simulink model "FDIBenchMark_BLW_test_b_1025"  (Simulink 7.3)
settings: Solver=ode45  StartTime=0  StopTime=4400  FixedStep=Ts  RelTol=1e-12
InitFcn:
  | FDIBenchMarkData
  | initialization
values from neighbouring files (symbols this model uses):
  a = 2.2    [FDIBenchMarkData.m]
  Addt = [-(B_dt+B_r)/J_r B_dt/N_g/J_r -K_dt/J_r; eta_dt*B_dt/N_g/J_g -(eta_dt*B_dt/N_g^2+B_g)/J_g eta_dt*K_dt/N_g/J_g; 1 -1/N_g 0]    [FDIBenchMarkData.m]
  Addt2 = [-(B_dt+B_r)/J_r B_dt/N_g/J_r -K_dt/J_r; eta_dt2*B_dt/N_g/J_g -(eta_dt2*B_dt/N_g^2+B_g)/J_g eta_dt2*K_dt/N_g/J_g; 1 -1/N_g 0]    [FDIBenchMarkData.m]
  alpha = 0.1    [FDIBenchMarkData.m]
  alpha_gc = 1/20e-3    (= 50)    [FDIBenchMarkData.m]
  Apb_E = Apb+A_f    [initialization.m]
  Bddt = [1/J_r 0; 0 -1/J_g;0 0]    [FDIBenchMarkData.m]
  Bddt2 = [1/J_r 0; 0 -1/J_g;0 0]    [FDIBenchMarkData.m]
  Cddt = [1 0 0;0 1 0]    [FDIBenchMarkData.m]
  Constant_Beta_1_m1 = 5    [FDIBenchMarkData.m]
  Constant_Beta_3_m1 = 10    [FDIBenchMarkData.m]
  Constant_Omega_r_m1 = 1.4    [FDIBenchMarkData.m]
  Constant_tau_gc = 100    [FDIBenchMarkData.m]
  eta_gc = 0.98    [FDIBenchMarkData.m]
  Gain_Beta_2_m2 = 1.2    [FDIBenchMarkData.m]
  Gain_Omega_r_m2 = 1.1    [FDIBenchMarkData.m]
  H = 87    [FDIBenchMarkData.m]
  k = 4.7    [FDIBenchMarkData.m]
  K_i = 1    [FDIBenchMarkData.m]
  K_opt = .5* rho* pi*R^2*eta_dt*R^3*0.4554/(N_g*8)^3    (= 1.21708013189)    [FDIBenchMarkData.m]
  K_p = 4    [FDIBenchMarkData.m]
  L = Length_scale    (= 600)    [FDIBenchMarkData.m]
  Lpb = Lpb'    [initialization.m]
  Lpb_FD = Lpb_FD'    [initialization.m]
  m = 1+alpha*(alpha-1)*R^2/(8*H^2)    (= 0.995085835315)    [FDIBenchMarkData.m]
  m_vw = 1.5    [FDIBenchMarkData.m]
  Omega_delta = 15    [FDIBenchMarkData.m]
  omega_n = 11.11    [FDIBenchMarkData.m]
  Omega_nom = 162    [FDIBenchMarkData.m]
  P_r = 4.8e6    (= 4800000)    [FDIBenchMarkData.m]
  R = 57.5    [FDIBenchMarkData.m]
  r = D_rotor/2    (= 57.5)    [FDIBenchMarkData.m]
  r0 = 1.5    [FDIBenchMarkData.m]
  rho = 1.225    [FDIBenchMarkData.m]
  seed = ceil(seed)    [FDIBenchMarkData.m]
  T_sample = 0.05    [FDIBenchMarkData.m]
  Ts = 1/100    (= 0.01)    [FDIBenchMarkData.m]
  turb_int = Turbulence_intensity    (= 12)    [FDIBenchMarkData.m]
  turbulence_seeds = [seed1 seed2]    [FDIBenchMarkData.m]
  xi = 0.6    [FDIBenchMarkData.m]
undefined symbols (not defined in the file or in its folder): Apb, Apb1, Apb2, Bpb, Bpb1, Bpb2, Cpb, Cpb1, Cpb2, Cq, DiscIntNeverNeededParam, u0
libraries: simulink x30
(part 1 of 2)
settings Model: Creator=peodg  LastModifiedBy=WSUadm
settings SolverCC: MaxConsecutiveZCs=1e6
settings OptimizationCC: InitFltsAndDblsToZero=on

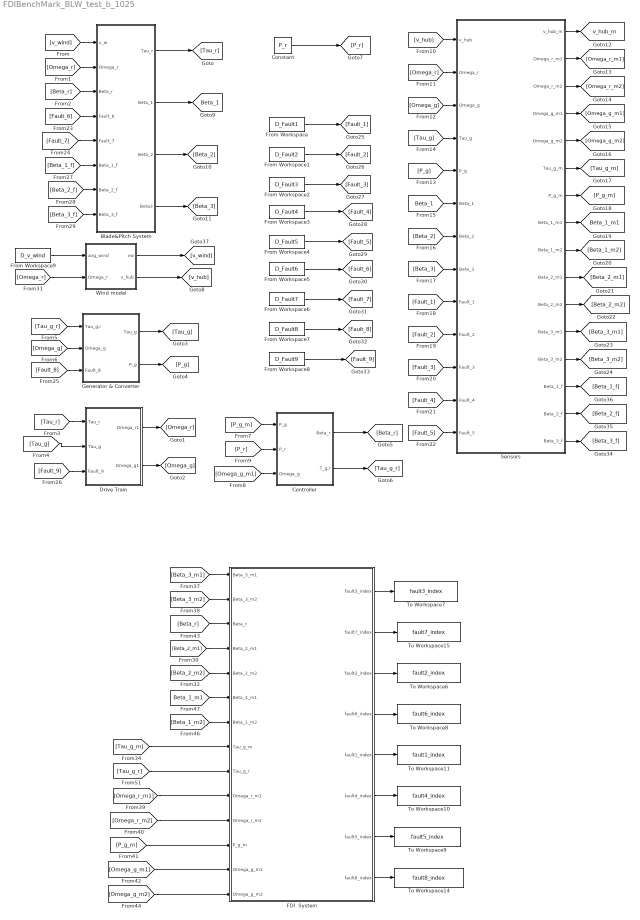
== system FDIBenchMark_BLW_test_b_1025 ==
  Blade&Pitch System : Subsystem
  Constant : Constant  Value=P_r  OutDataType=sfix(16)  OutScaling=2^0
  Controller : Subsystem
  Drive Train : Subsystem
  FDI  System : Subsystem
  From Workspace : FromWorkspace  VariableName=D_Fault1  SampleTime=Ts
  From Workspace1 : FromWorkspace  VariableName=D_Fault2  SampleTime=Ts
  From Workspace2 : FromWorkspace  VariableName=D_Fault3  SampleTime=Ts
  From Workspace3 : FromWorkspace  VariableName=D_Fault4  SampleTime=Ts
  From Workspace4 : FromWorkspace  VariableName=D_Fault5  SampleTime=Ts
  From Workspace5 : FromWorkspace  VariableName=D_Fault6  SampleTime=Ts
  From Workspace6 : FromWorkspace  VariableName=D_Fault7  SampleTime=Ts
  From Workspace7 : FromWorkspace  VariableName=D_Fault8  SampleTime=Ts
  From Workspace8 : FromWorkspace  VariableName=D_Fault9  SampleTime=Ts
  From Workspace9 : FromWorkspace  VariableName=D_v_wind
  Generator & Converter : Subsystem
  Sensors : Subsystem
  To Workspace10 : ToWorkspace  VariableName=fault4_index  SampleTime=-1  SaveFormat=Array
  To Workspace11 : ToWorkspace  VariableName=fault1_index  SampleTime=-1  SaveFormat=Array
  To Workspace14 : ToWorkspace  VariableName=fault8_index  SampleTime=-1  SaveFormat=Array
  To Workspace15 : ToWorkspace  VariableName=fault7_index  SampleTime=-1  SaveFormat=Array
  To Workspace6 : ToWorkspace  VariableName=fault2_index  SampleTime=-1  SaveFormat=Array
  To Workspace7 : ToWorkspace  VariableName=fault3_index  SampleTime=-1  SaveFormat=Array
  To Workspace8 : ToWorkspace  VariableName=fault6_index  SampleTime=-1  SaveFormat=Array
  To Workspace9 : ToWorkspace  VariableName=fault5_index  SampleTime=-1  SaveFormat=Array
  Wind model : Subsystem
  tag scope: Beta_1=global, Beta_1_m1=global, v_hub_m=global
  wires:
  [v_wind] -> Blade&Pitch System/1(v_w)
  [Omega_r] -> Blade&Pitch System/2(Omega_r)
  [Beta_r] -> Blade&Pitch System/3(Beta_r)
  [Tau_r] -> Drive Train/1(Tau_r)
  [Tau_g] -> Drive Train/2(Tau_g)
  Drive Train/1(Omega_r1) -> [Omega_r]
  [Tau_g_r] -> Generator & Converter/1(Tau_g,r)
  [Omega_g] -> Generator & Converter/2(Omega_g)
  Generator & Converter/1(Tau_g) -> [Tau_g]
  Generator & Converter/2(P_g) -> [P_g]
  [P_g_m] -> Controller/1(P_g)
  [Omega_g_m1] -> Controller/3(Omega_g)
  Controller/2(T_g,r) -> [Tau_g_r]
  [P_r] -> Controller/2(P_r)
  Constant/1 -> [P_r]
  Sensors/1(v_hub_m) -> [v_hub_m]
  Sensors/2(Omega_r_m1) -> [Omega_r_m1]
  Sensors/3(Omega_r_m2) -> [Omega_r_m2]
  Sensors/4(Omega_g_m1) -> [Omega_g_m1]
  Sensors/5(Omega_g_m2) -> [Omega_g_m2]
  Sensors/6(Tau_g_m) -> [Tau_g_m]
  Sensors/7(P_g_m) -> [P_g_m]
  Sensors/8(Beta_1_m1) -> [Beta_1_m1]
  Sensors/9(Beta_1_m2) -> [Beta_1_m2]
  Sensors/10(Beta_2_m1) -> [Beta_2_m1]
  Sensors/11(Beta_2_m2) -> [Beta_2_m2]
  Sensors/12(Beta_3_m1) -> [Beta_3_m1]
  Sensors/13(Beta_3_m2) -> [Beta_3_m2]
  [v_hub] -> Sensors/1(v_hub)
  [Omega_r] -> Sensors/2(Omega_r)
  [Omega_g] -> Sensors/3(Omega_g)
  [Tau_g] -> Sensors/4(Tau_g)
  [P_g] -> Sensors/5(P_g)
  [Beta_1] -> Sensors/6(Beta_1)
  [Beta_2] -> Sensors/7(Beta_2)
  [Beta_3] -> Sensors/8(Beta_3)
  [Fault_1] -> Sensors/9(Fault_1)
  [Fault_2] -> Sensors/10(Fault_2)
  [Fault_3] -> Sensors/11(Fault_3)
  [Fault_4] -> Sensors/12(Fault_4)
  [Fault_5] -> Sensors/13(Fault_5)
  [Fault_6] -> Blade&Pitch System/4(Fault_6)
  [Fault_7] -> Blade&Pitch System/5(Fault_7)
  [Fault_8] -> Generator & Converter/3(Fault_8)
  [Fault_9] -> Drive Train/3(Fault_9)
  From Workspace8/1 -> [Fault_9]
  From Workspace7/1 -> [Fault_8]
  From Workspace6/1 -> [Fault_7]
  From Workspace5/1 -> [Fault_6]
  From Workspace4/1 -> [Fault_5]
  From Workspace3/1 -> [Fault_4]
  From Workspace2/1 -> [Fault_3]
  From Workspace1/1 -> [Fault_2]
  From Workspace/1 -> [Fault_1]
  Drive Train/2(Omega_g1) -> [Omega_g]
  Sensors/16(Beta_3_f) -> [Beta_3_f]
  Sensors/15(Beta_2_f) -> [Beta_2_f]
  Sensors/14(Beta_1_f) -> [Beta_1_f]
  [Beta_1_f] -> Blade&Pitch System/6(Beta_1_f)
  [Beta_2_f] -> Blade&Pitch System/7(Beta_2_f)
  [Beta_3_f] -> Blade&Pitch System/8(Beta_3_f)
  Blade&Pitch System/4(Beta3) -> [Beta_3]
  Blade&Pitch System/3(Beta_2) -> [Beta_2]
  Blade&Pitch System/2(Beta_1) -> [Beta_1]
  Blade&Pitch System/1(Tau_r) -> [Tau_r]
  Wind model/1(vw) -> [v_wind]
  Wind model/2(v_hub) -> [v_hub]
  [Omega_r] -> Wind model/2(Omega_r)
  From Workspace9/1 -> Wind model/1(avg_wind)
  Controller/1(Beta_r) -> [Beta_r]
  FDI  System/1(fault3_index) -> To Workspace7/1
  FDI  System/2(fault7_index) -> To Workspace15/1
  [Beta_3_m1] -> FDI  System/1(Beta_3_m1)
  [Beta_3_m2] -> FDI  System/2(Beta_3_m2)
  FDI  System/3(fault2_index) -> To Workspace6/1
  FDI  System/4(fault6_index) -> To Workspace8/1
  [Beta_r] -> FDI  System/3(Beta_r)
  [Beta_2_m1] -> FDI  System/4(Beta_2_m1)
  [Beta_2_m2] -> FDI  System/5(Beta_2_m2)
  FDI  System/5(fault1_index) -> To Workspace11/1
  [Beta_1_m2] -> FDI  System/7(Beta_1_m2)
  [Beta_1_m1] -> FDI  System/6(Beta_1_m1)
  FDI  System/6(fault4_index) -> To Workspace10/1
  FDI  System/7(fault5_index) -> To Workspace9/1
  FDI  System/8(fault8_index) -> To Workspace14/1
  [Omega_g_m1] -> FDI  System/13(Omega_g_m1)
  [Omega_r_m1] -> FDI  System/10(Omega_r_m1)
  [Tau_g_m] -> FDI  System/8(Tau_g_m)
  [Omega_r_m2] -> FDI  System/11(Omega_r_m2)
  [Tau_g_r] -> FDI  System/9(Tau_g_r)
  [P_g_m] -> FDI  System/12(P_g_m)
  [Omega_g_m2] -> FDI  System/14(Omega_g_m2)

== system FDIBenchMark_BLW_test_b_1025/Blade&Pitch System ==
  v_w : Inport  OutDataType=sfix(16)  OutScaling=2^0
  Omega_r : Inport  Port=2  OutDataType=sfix(16)  OutScaling=2^0
  Beta_r : Inport  Port=3  OutDataType=sfix(16)  OutScaling=2^0
  Fault_6 : Inport  Port=4  OutDataType=sfix(16)  OutScaling=2^0
  Fault_7 : Inport  Port=5  OutDataType=sfix(16)  OutScaling=2^0
  Beta_1_f : Inport  Port=6  OutDataType=sfix(16)  OutScaling=2^0
  Beta_2_f : Inport  Port=7  OutDataType=sfix(16)  OutScaling=2^0
  Beta_3_f : Inport  Port=8  OutDataType=sfix(16)  OutScaling=2^0
  Add : Sum  OutDataType=sfix(16)  OutScaling=2^-10
  Add1 : Sum  OutDataType=sfix(16)  OutScaling=2^-10
  Add2 : Sum  OutDataType=sfix(16)  OutScaling=2^-10
  Pitch Systems : Subsystem
  Subsystem : Subsystem
  To Workspace6 : ToWorkspace  VariableName=Tau_r  SampleTime=-1  SaveFormat=Array
  Tau_r : Outport  OutDataType=sfix(16)  OutScaling=2^0
  Beta_1 : Outport  Port=2  OutDataType=sfix(16)  OutScaling=2^0
  Beta_2 : Outport  Port=3  OutDataType=sfix(16)  OutScaling=2^0
  Beta3 : Outport  Port=4  OutDataType=sfix(16)  OutScaling=2^0
  wires:
  Pitch Systems/1(Beta_1) -> Subsystem/3(Beta_1), Beta_1/1
  Pitch Systems/2(Beta_2) -> Subsystem/4(Beta_2), Beta_2/1
  Pitch Systems/3(Beta_3) -> Subsystem/5(Beta_3), Beta3/1
  Subsystem/1(Tau_r) -> Tau_r/1, To Workspace6/1
  v_w/1 -> Subsystem/1(v_w)
  Omega_r/1 -> Subsystem/2(Omega_r)
  Fault_6/1 -> Pitch Systems/4(Fault_6)
  Fault_7/1 -> Pitch Systems/5(Fault_7)
  Add/1 -> Pitch Systems/3(Beta_r3)
  Add1/1 -> Pitch Systems/1(Beta_r1)
  Add2/1 -> Pitch Systems/2(Beta_r2)
  Beta_3_f/1 -> Add/2
  Beta_2_f/1 -> Add2/2
  Beta_1_f/1 -> Add1/2
  Beta_r/1 -> Add1/1, Add2/1, Add/1

== system FDIBenchMark_BLW_test_b_1025/Controller ==
  P_g : Inport  OutDataType=sfix(16)  OutScaling=2^0
  P_r : Inport  Port=2  OutDataType=sfix(16)  OutScaling=2^0
  Omega_g : Inport  Port=3  OutDataType=sfix(16)  OutScaling=2^0
  Constant : Constant  Value=Omega_nom  OutDataType=sfix(16)  OutScaling=2^0
  Constant1 : Constant  Value=Omega_delta  OutDataType=sfix(16)  OutScaling=2^0
  Embedded MATLAB Function : Stateflow chart
  Subsystem : Subsystem
  Subsystem1 : Subsystem
  Switch : Switch  Threshold=.5  OutDataType=sfix(16)  OutScaling=2^0
  Switch1 : Switch  Threshold=.5  OutDataType=sfix(16)  OutScaling=2^0
  Unit Delay : UnitDelay  SampleTime=Ts
  Zero-Order Hold : ZeroOrderHold  SampleTime=Ts
  Zero-Order Hold1 : ZeroOrderHold  SampleTime=Ts
  Zero-Order Hold2 : ZeroOrderHold  SampleTime=Ts
  Beta_r : Outport  OutDataType=sfix(16)  OutScaling=2^0
  T_g,r : Outport  Port=2  OutDataType=sfix(16)  OutScaling=2^0
  wires:
  Embedded MATLAB Function/1(ControlZone) -> Unit Delay/1, Switch/2, Switch1/2
  Unit Delay/1 -> Embedded MATLAB Function/4(LastControlZone)
  P_g/1 -> Zero-Order Hold/1
  P_r/1 -> Zero-Order Hold1/1
  Omega_g/1 -> Zero-Order Hold2/1
  Switch/1 -> Beta_r/1
  Switch1/1 -> T_g,r/1
  Subsystem1/1(Beta_r) -> Switch/1
  Subsystem/1(Beta_r) -> Switch/3
  Subsystem1/2(Tau_g,r) -> Switch1/1
  Subsystem/2(T_g,r) -> Switch1/3
  Constant/1 -> Embedded MATLAB Function/5(Omega_nom)
  Constant1/1 -> Embedded MATLAB Function/6(Omega_delta)
  Zero-Order Hold/1 -> Embedded MATLAB Function/1(P_g)
  Zero-Order Hold1/1 -> Embedded MATLAB Function/2(P_r), Subsystem1/1(P_r)
  Zero-Order Hold2/1 -> Embedded MATLAB Function/3(Omega_g), Subsystem1/2(Omega_g), Subsystem/1(Omega_g)

== system FDIBenchMark_BLW_test_b_1025/Drive Train ==
  Tau_r : Inport  OutDataType=sfix(16)  OutScaling=2^0
  Tau_g : Inport  Port=2  OutDataType=sfix(16)  OutScaling=2^0
  Fault_9 : Inport  Port=3  OutDataType=sfix(16)  OutScaling=2^0
  Add : Sum  OutDataType=sfix(16)  OutScaling=2^-10
  Demux1 : Demux  Outputs=2
  Gain : Gain  Gain=Addt  Multiplication=Matrix(K*u)  ParameterDataType=sfix(16)  ParameterScaling=2^0  OutDataType=sfix(16)  OutScaling=2^0
  Gain1 : Gain  Gain=Bddt  Multiplication=Matrix(K*u)  ParameterDataType=sfix(16)  ParameterScaling=2^0  OutDataType=sfix(16)  OutScaling=2^0
  Gain2 : Gain  Gain=Cddt  Multiplication=Matrix(K*u)  ParameterDataType=sfix(16)  ParameterScaling=2^0  OutDataType=sfix(16)  OutScaling=2^0
  Gain3 : Gain  Gain=Addt2  Multiplication=Matrix(K*u)  ParameterDataType=sfix(16)  ParameterScaling=2^0  OutDataType=sfix(16)  OutScaling=2^0
  Gain4 : Gain  Gain=Bddt2  Multiplication=Matrix(K*u)  ParameterDataType=sfix(16)  ParameterScaling=2^0  OutDataType=sfix(16)  OutScaling=2^0
  Integrator : Integrator  InitialCondition=[1 100 0]
  Mux : Mux  Inputs=2
  Switch1 : Switch  Threshold=0.5  OutDataType=sfix(16)  OutScaling=2^0
  Switch2 : Switch  Threshold=0.5  OutDataType=sfix(16)  OutScaling=2^0
  Omega_r1 : Outport  OutDataType=sfix(16)  OutScaling=2^0
  Omega_g1 : Outport  Port=2  OutDataType=sfix(16)  OutScaling=2^0
  wires:
  Tau_r/1 -> Mux/1
  Tau_g/1 -> Mux/2
  Integrator/1 -> Gain/1, Gain3/1, Gain2/1
  Add/1 -> Integrator/1
  Switch1/1 -> Add/1
  Gain1/1 -> Switch1/1
  Gain4/1 -> Switch1/3
  Gain/1 -> Switch2/1
  Gain3/1 -> Switch2/3
  Switch2/1 -> Add/2
  Demux1/1 -> Omega_r1/1
  Demux1/2 -> Omega_g1/1
  Gain2/1 -> Demux1/1
  Fault_9/1 -> Switch1/2, Switch2/2
  Mux/1 -> Gain1/1, Gain4/1

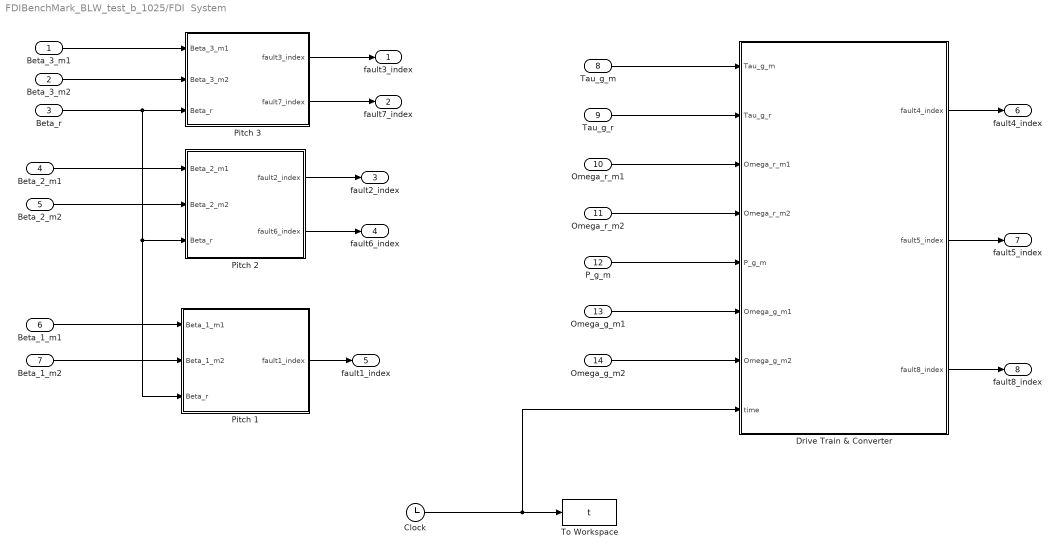
== system FDIBenchMark_BLW_test_b_1025/FDI  System ==
  Beta_3_m1 : Inport  OutDataType=fixdt(1, 16)  OutScaling=2^0
  Beta_3_m2 : Inport  Port=2  OutDataType=fixdt(1, 16)  OutScaling=2^0
  Beta_r : Inport  Port=3  OutDataType=fixdt(1, 16)  OutScaling=2^0
  Beta_2_m1 : Inport  Port=4  OutDataType=fixdt(1, 16)  OutScaling=2^0
  Beta_2_m2 : Inport  Port=5  OutDataType=fixdt(1, 16)  OutScaling=2^0
  Beta_1_m1 : Inport  Port=6  OutDataType=fixdt(1, 16)  OutScaling=2^0
  Beta_1_m2 : Inport  Port=7  OutDataType=fixdt(1, 16)  OutScaling=2^0
  Tau_g_m : Inport  Port=8  OutDataType=fixdt(1, 16)  OutScaling=2^0
  Tau_g_r : Inport  Port=9  OutDataType=fixdt(1, 16)  OutScaling=2^0
  Omega_r_m1 : Inport  Port=10  OutDataType=fixdt(1, 16)  OutScaling=2^0
  Omega_r_m2 : Inport  Port=11  OutDataType=fixdt(1, 16)  OutScaling=2^0
  P_g_m : Inport  Port=12  OutDataType=fixdt(1, 16)  OutScaling=2^0
  Omega_g_m1 : Inport  Port=13  OutDataType=fixdt(1, 16)  OutScaling=2^0
  Omega_g_m2 : Inport  Port=14  OutDataType=fixdt(1, 16)  OutScaling=2^0
  Clock : Clock
      settings: Decimation=10
  Drive Train & Converter : Subsystem
  Pitch 1 : Subsystem
  Pitch 2 : Subsystem
  Pitch 3 : Subsystem
  To Workspace : ToWorkspace  VariableName=t  SampleTime=-1  SaveFormat=Array
  fault3_index : Outport  OutDataType=fixdt(1, 16)  OutScaling=2^0
  fault7_index : Outport  Port=2  OutDataType=fixdt(1, 16)  OutScaling=2^0
  fault2_index : Outport  Port=3  OutDataType=fixdt(1, 16)  OutScaling=2^0
  fault6_index : Outport  Port=4  OutDataType=fixdt(1, 16)  OutScaling=2^0
  fault1_index : Outport  Port=5  OutDataType=fixdt(1, 16)  OutScaling=2^0
  fault4_index : Outport  Port=6  OutDataType=fixdt(1, 16)  OutScaling=2^0
  fault5_index : Outport  Port=7  OutDataType=fixdt(1, 16)  OutScaling=2^0
  fault8_index : Outport  Port=8  OutDataType=fixdt(1, 16)  OutScaling=2^0
  wires:
  Pitch 3/1(fault3_index) -> fault3_index/1
  Pitch 3/2(fault7_index) -> fault7_index/1
  Beta_3_m1/1 -> Pitch 3/1(Beta_3_m1)
  Beta_3_m2/1 -> Pitch 3/2(Beta_3_m2)
  Beta_r/1 -> Pitch 3/3(Beta_r), Pitch 2/3(Beta_r), Pitch 1/3(Beta_r)
  Pitch 2/1(fault2_index) -> fault2_index/1
  Pitch 2/2(fault6_index) -> fault6_index/1
  Beta_2_m1/1 -> Pitch 2/1(Beta_2_m1)
  Beta_2_m2/1 -> Pitch 2/2(Beta_2_m2)
  Beta_1_m1/1 -> Pitch 1/1(Beta_1_m1)
  Beta_1_m2/1 -> Pitch 1/2(Beta_1_m2)
  Pitch 1/1(fault1_index) -> fault1_index/1
  Drive Train & Converter/1(fault4_index) -> fault4_index/1
  Drive Train & Converter/2(fault5_index) -> fault5_index/1
  Drive Train & Converter/3(fault8_index) -> fault8_index/1
  Tau_g_m/1 -> Drive Train & Converter/1(Tau_g_m)
  Tau_g_r/1 -> Drive Train & Converter/2(Tau_g_r)
  Omega_r_m1/1 -> Drive Train & Converter/3(Omega_r_m1)
  Omega_r_m2/1 -> Drive Train & Converter/4(Omega_r_m2)
  P_g_m/1 -> Drive Train & Converter/5(P_g_m)
  Omega_g_m1/1 -> Drive Train & Converter/6(Omega_g_m1)
  Omega_g_m2/1 -> Drive Train & Converter/7(Omega_g_m2)
  Clock/1 -> To Workspace/1, Drive Train & Converter/8(time)

== system FDIBenchMark_BLW_test_b_1025/Generator & Converter ==
  Tau_g,r : Inport  OutDataType=sfix(16)  OutScaling=2^0
  Omega_g : Inport  Port=2  OutDataType=sfix(16)  OutScaling=2^0
  Fault_8 : Inport  Port=3  OutDataType=sfix(16)  OutScaling=2^0
  Bias : Bias  Bias=Constant_tau_gc
  Divide : Product  Inputs=**  OutDataType=sfix(16)  OutScaling=2^-10
  Gain : Gain  Gain=eta_gc  ParameterDataType=sfix(16)  ParameterScaling=2^0  OutDataType=sfix(16)  OutScaling=2^0
  Switch : Switch  Threshold=0.5  OutDataType=sfix(16)  OutScaling=2^0
  Transfer Fcn : TransferFcn  Numerator=[alpha_gc]  Denominator=[1 alpha_gc]
  Tau_g : Outport  OutDataType=sfix(16)  OutScaling=2^0
  P_g : Outport  Port=2  OutDataType=sfix(16)  OutScaling=2^0
  wires:
  Tau_g,r/1 -> Transfer Fcn/1
  Gain/1 -> P_g/1
  Divide/1 -> Gain/1
  Omega_g/1 -> Divide/2
  Transfer Fcn/1 -> Bias/1, Switch/1
  Fault_8/1 -> Switch/2
  Switch/1 -> Divide/1, Tau_g/1
  Bias/1 -> Switch/3

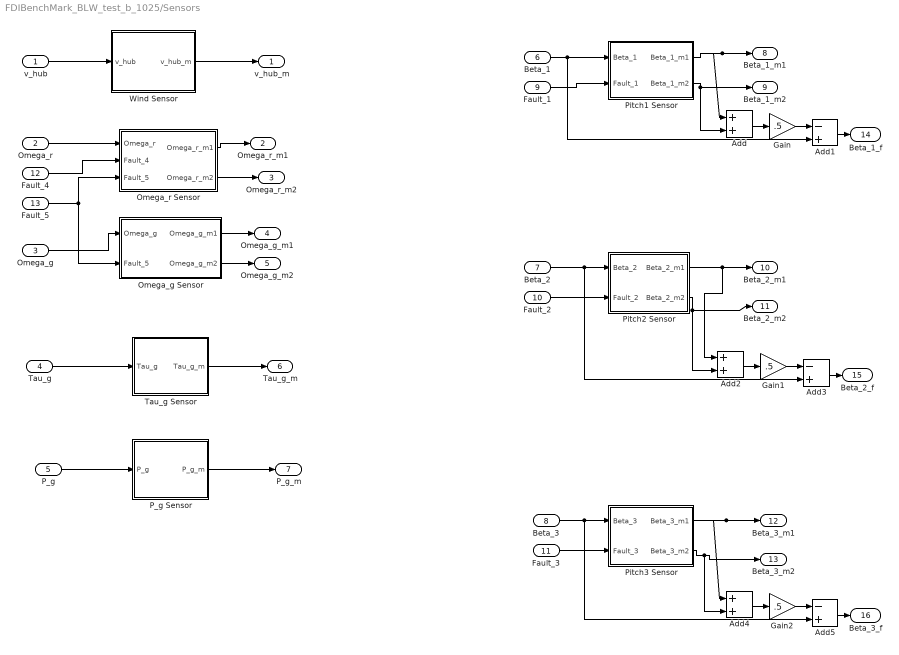
== system FDIBenchMark_BLW_test_b_1025/Sensors ==
  v_hub : Inport  OutDataType=sfix(16)  OutScaling=2^0
  Omega_r : Inport  Port=2  OutDataType=sfix(16)  OutScaling=2^0
  Omega_g : Inport  Port=3  OutDataType=sfix(16)  OutScaling=2^0
  Tau_g : Inport  Port=4  OutDataType=sfix(16)  OutScaling=2^0
  P_g : Inport  Port=5  OutDataType=sfix(16)  OutScaling=2^0
  Beta_1 : Inport  Port=6  OutDataType=sfix(16)  OutScaling=2^0
  Beta_2 : Inport  Port=7  OutDataType=sfix(16)  OutScaling=2^0
  Beta_3 : Inport  Port=8  OutDataType=sfix(16)  OutScaling=2^0
  Fault_1 : Inport  Port=9  OutDataType=sfix(16)  OutScaling=2^0
  Fault_2 : Inport  Port=10  OutDataType=sfix(16)  OutScaling=2^0
  Fault_3 : Inport  Port=11  OutDataType=sfix(16)  OutScaling=2^0
  Fault_4 : Inport  Port=12  OutDataType=sfix(16)  OutScaling=2^0
  Fault_5 : Inport  Port=13  OutDataType=sfix(16)  OutScaling=2^0
  Add : Sum  OutDataType=sfix(16)  OutScaling=2^-10
  Add1 : Sum  Inputs=-+  OutDataType=sfix(16)  OutScaling=2^-10
  Add2 : Sum  OutDataType=sfix(16)  OutScaling=2^-10
  Add3 : Sum  Inputs=-+  OutDataType=sfix(16)  OutScaling=2^-10
  Add4 : Sum  OutDataType=sfix(16)  OutScaling=2^-10
  Add5 : Sum  Inputs=-+  OutDataType=sfix(16)  OutScaling=2^-10
  Gain : Gain  Gain=.5  ParameterDataType=sfix(16)  ParameterScaling=2^0  OutDataType=sfix(16)  OutScaling=2^0
  Gain1 : Gain  Gain=.5  ParameterDataType=sfix(16)  ParameterScaling=2^0  OutDataType=sfix(16)  OutScaling=2^0
  Gain2 : Gain  Gain=.5  ParameterDataType=sfix(16)  ParameterScaling=2^0  OutDataType=sfix(16)  OutScaling=2^0
  Omega_g Sensor : Subsystem
  Omega_r Sensor : Subsystem
  P_g Sensor : Subsystem
  Pitch1 Sensor : Subsystem
  Pitch2 Sensor : Subsystem
  Pitch3 Sensor : Subsystem
  Tau_g Sensor : Subsystem
  Wind Sensor : Subsystem
  v_hub_m : Outport  OutDataType=sfix(16)  OutScaling=2^0
  Omega_r_m1 : Outport  Port=2  OutDataType=sfix(16)  OutScaling=2^0
  Omega_r_m2 : Outport  Port=3  OutDataType=sfix(16)  OutScaling=2^0
  Omega_g_m1 : Outport  Port=4  OutDataType=sfix(16)  OutScaling=2^0
  Omega_g_m2 : Outport  Port=5  OutDataType=sfix(16)  OutScaling=2^0
  Tau_g_m : Outport  Port=6  OutDataType=sfix(16)  OutScaling=2^0
  P_g_m : Outport  Port=7  OutDataType=sfix(16)  OutScaling=2^0
  Beta_1_m1 : Outport  Port=8  OutDataType=sfix(16)  OutScaling=2^0
  Beta_1_m2 : Outport  Port=9  OutDataType=sfix(16)  OutScaling=2^0
  Beta_2_m1 : Outport  Port=10  OutDataType=sfix(16)  OutScaling=2^0
  Beta_2_m2 : Outport  Port=11  OutDataType=sfix(16)  OutScaling=2^0
  Beta_3_m1 : Outport  Port=12  OutDataType=sfix(16)  OutScaling=2^0
  Beta_3_m2 : Outport  Port=13  OutDataType=sfix(16)  OutScaling=2^0
  Beta_1_f : Outport  Port=14  OutDataType=sfix(16)  OutScaling=2^0
  Beta_2_f : Outport  Port=15  OutDataType=sfix(16)  OutScaling=2^0
  Beta_3_f : Outport  Port=16  OutDataType=sfix(16)  OutScaling=2^0
  wires:
  Wind Sensor/1(v_hub_m) -> v_hub_m/1
  v_hub/1 -> Wind Sensor/1(v_hub)
  Omega_r/1 -> Omega_r Sensor/1(Omega_r)
  Omega_r Sensor/1(Omega_r_m1) -> Omega_r_m1/1
  Omega_r Sensor/2(Omega_r_m2) -> Omega_r_m2/1
  Omega_g/1 -> Omega_g Sensor/1(Omega_g)
  Omega_g Sensor/1(Omega_g_m1) -> Omega_g_m1/1
  Omega_g Sensor/2(Omega_g_m2) -> Omega_g_m2/1
  Tau_g/1 -> Tau_g Sensor/1(Tau_g)
  Tau_g Sensor/1(Tau_g_m) -> Tau_g_m/1
  P_g/1 -> P_g Sensor/1(P_g)
  P_g Sensor/1(P_g_m) -> P_g_m/1
  Beta_1/1 -> Pitch1 Sensor/1(Beta_1), Add1/2
  Pitch1 Sensor/1(Beta_1_m1) -> Beta_1_m1/1, Add/1
  Pitch1 Sensor/2(Beta_1_m2) -> Beta_1_m2/1, Add/2
  Beta_2/1 -> Pitch2 Sensor/1(Beta_2), Add3/2
  Pitch2 Sensor/1(Beta_2_m1) -> Beta_2_m1/1, Add2/1
  Pitch2 Sensor/2(Beta_2_m2) -> Beta_2_m2/1, Add2/2
  Beta_3/1 -> Pitch3 Sensor/1(Beta_3), Add5/2
  Pitch3 Sensor/1(Beta_3_m1) -> Beta_3_m1/1, Add4/1
  Pitch3 Sensor/2(Beta_3_m2) -> Beta_3_m2/1, Add4/2
  Fault_1/1 -> Pitch1 Sensor/2(Fault_1)
  Fault_2/1 -> Pitch2 Sensor/2(Fault_2)
  Fault_3/1 -> Pitch3 Sensor/2(Fault_3)
  Fault_4/1 -> Omega_r Sensor/2(Fault_4)
  Fault_5/1 -> Omega_r Sensor/3(Fault_5), Omega_g Sensor/2(Fault_5)
  Add/1 -> Gain/1
  Gain/1 -> Add1/1
  Add1/1 -> Beta_1_f/1
  Add2/1 -> Gain1/1
  Gain1/1 -> Add3/1
  Add3/1 -> Beta_2_f/1
  Add4/1 -> Gain2/1
  Gain2/1 -> Add5/1
  Add5/1 -> Beta_3_f/1

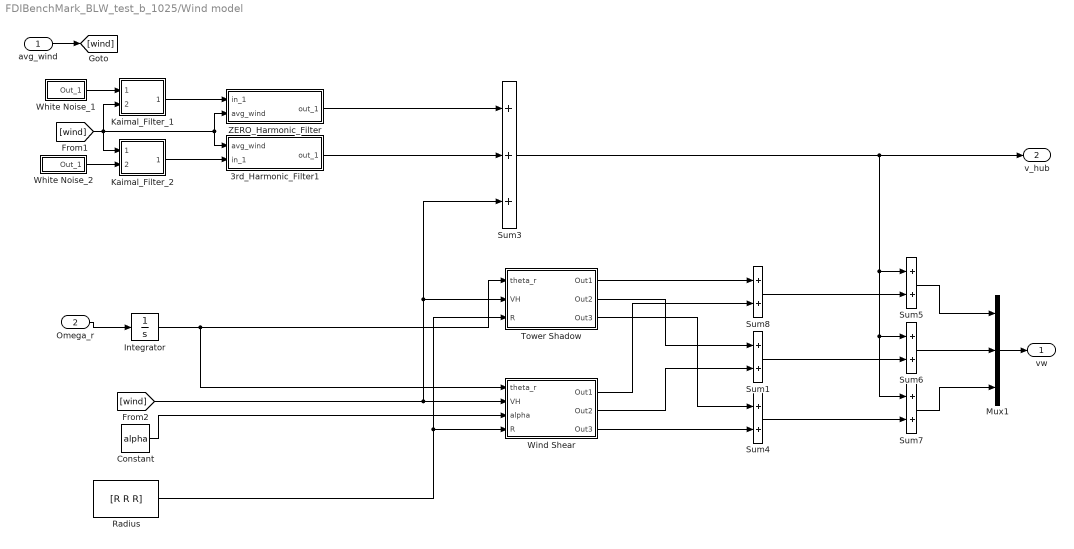
== system FDIBenchMark_BLW_test_b_1025/Wind model ==
  avg_wind : Inport  OutDataType=sfix(16)  OutScaling=2^0
  Omega_r : Inport  Port=2  OutDataType=sfix(16)  OutScaling=2^0
  3rd_Harmonic_Filter1 : Subsystem
  Constant : Constant  Value=alpha  OutDataType=sfix(16)  OutScaling=2^0
  Integrator : Integrator
  Kaimal_Filter_1 : Subsystem
  Kaimal_Filter_2 : Subsystem
  Mux1 : Mux  Inputs=3
  Radius : Constant  Value=[R R R]  OutDataType=sfix(16)  OutScaling=2^0
  Sum{1,4..8} (6 alike) : Sum  OutDataType=sfix(16)  OutScaling=2^0  SaturateOnIntegerOverflow=on  InputSameDT=on  OutDataTypeStr=Inherit: Same as first input
  Sum3 : Sum  Inputs=+++  OutDataType=sfix(16)  OutScaling=2^0  SaturateOnIntegerOverflow=on  InputSameDT=on  OutDataTypeStr=Inherit: Same as first input
  Tower Shadow : Subsystem
  White Noise_1 : Subsystem  mask(Continuous White Noise.){Cov=[1], Ts=T_sample, seed=turbulence_seeds(1)}
      mask prompts: Cov "Noise Power:"; Ts "Sample Time:"
      mask help:
      | White noise for continuous (s-domain) systems.
      | Band-limited using zero-order-hold.
      mask init:
      | r = rand(1,12); r2 = [r(1),r;r,r(12)]; t =[1:13;1:13];
      mask Help: Implemented using white noise into Zero-Order Hold block. The seed and power can be vectors of the same length to produce a vector of white noise sources. For faster simulation, set sample time to the highest value possible but in accordance with the fastest dynamics of system.
      mask Display: plot(t(:),r2(:))
  White Noise_2 : Subsystem  mask(Continuous White Noise.){@1=[1], @2=T_sample, @3=turbulence_seeds(2)}
      mask prompts: @1 "Noise Power:"; @2 "Sample Time:"; @3 "Seed"
      mask help:
      | White noise for continuous (s-domain) systems.
      | Band-limited using zero-order-hold.
      mask init:
      | Cov = @1; Ts = @2; seed = @3; r = rand(1,12); r2 = [r(1),r;r,r(12)]; t =[1:13;1:13];
      mask Help: Implemented using white noise into Zero-Order Hold block. The seed and power can be vectors of the same length to produce a vector of white noise sources. For faster simulation, set sample time to the highest value possible but in accordance with the fastest dynamics of system.
      mask Display: plot(t(:),r2(:))
  Wind Shear : Subsystem
  ZERO_Harmonic_Filter : Subsystem
  vw : Outport  OutDataType=sfix(16)  OutScaling=2^0  InitialOutput=[u0]
  v_hub : Outport  Port=2  OutDataType=sfix(16)  OutScaling=2^0  InitialOutput=[u0]
  wires:
  [wind] -> 3rd_Harmonic_Filter1/1(avg_wind), ZERO_Harmonic_Filter/2(avg_wind), Kaimal_Filter_2/1(avg_wind), Kaimal_Filter_1/2(avg_wind)
  avg_wind/1 -> [wind]
  White Noise_2/1(Out_1) -> Kaimal_Filter_2/2(in_1)
  Kaimal_Filter_2/1(out_1) -> 3rd_Harmonic_Filter1/2(in_1)
  Kaimal_Filter_1/1(out_1) -> ZERO_Harmonic_Filter/1(in_1)
  White Noise_1/1(Out_1) -> Kaimal_Filter_1/1(in_1)
  [wind] -> Wind Shear/2(VH), Sum3/3, Tower Shadow/2(VH)
  Constant/1 -> Wind Shear/3(alpha)
  Radius/1 -> Wind Shear/4(R), Tower Shadow/3(R)
  Tower Shadow/1(Out1) -> Sum8/1
  Wind Shear/1(Out1) -> Sum8/2
  Tower Shadow/2(Out2) -> Sum1/1
  Wind Shear/2(Out2) -> Sum1/2
  Tower Shadow/3(Out3) -> Sum4/1
  Wind Shear/3(Out3) -> Sum4/2
  Sum8/1 -> Sum5/2
  Sum1/1 -> Sum6/2
  Sum4/1 -> Sum7/2
  Sum5/1 -> Mux1/1
  Sum6/1 -> Mux1/2
  Sum7/1 -> Mux1/3
  Mux1/1 -> vw/1
  Sum3/1 -> Sum6/1, Sum7/1, Sum5/1, v_hub/1
  3rd_Harmonic_Filter1/1(out_1) -> Sum3/2
  ZERO_Harmonic_Filter/1(out_1) -> Sum3/1
  Omega_r/1 -> Integrator/1
  Integrator/1 -> Tower Shadow/1(theta_r), Wind Shear/1(theta_r)

== system FDIBenchMark_BLW_test_b_1025/Blade&Pitch System/Pitch Systems ==
  Beta_r1 : Inport
  Beta_r2 : Inport  Port=2
  Beta_r3 : Inport  Port=3
  Fault_6 : Inport  Port=4
  Fault_7 : Inport  Port=5
  PitchSystem 1 : Subsystem
  PitchSystem 2 : Subsystem
  PitchSystem 3 : Subsystem
  Beta_1 : Outport
  Beta_2 : Outport  Port=2
  Beta_3 : Outport  Port=3
  wires:
  PitchSystem 1/1(Beta_1) -> Beta_1/1
  PitchSystem 2/1(Beta_2) -> Beta_2/1
  PitchSystem 3/1(Beta_3) -> Beta_3/1
  Fault_7/1 -> PitchSystem 3/2(Fault_7)
  Fault_6/1 -> PitchSystem 2/2(Fault_6)
  Beta_r3/1 -> PitchSystem 3/1(Beta_r)
  Beta_r2/1 -> PitchSystem 2/1(Beta_r)
  Beta_r1/1 -> PitchSystem 1/1(Beta_r)

== system FDIBenchMark_BLW_test_b_1025/Blade&Pitch System/Subsystem ==
  v_w : Inport
  Omega_r : Inport  Port=2
  Beta_1 : Inport  Port=3
  Beta_2 : Inport  Port=4
  Beta_3 : Inport  Port=5
  Add : Sum  Inputs=+++  OutDataType=sfix(16)  OutScaling=2^-10
  AeroDyn 1 : Subsystem
  AeroDyn 2 : Subsystem
  AeroDyn 3 : Subsystem
  Demux : Demux  Outputs=3
  Tau_r : Outport
  wires:
  Omega_r/1 -> AeroDyn 1/2(Omega_r), AeroDyn 2/2(Omega_r), AeroDyn 3/2(Omega_r)
  AeroDyn 1/1(Tau_r1) -> Add/1
  AeroDyn 2/1(Tau_r2) -> Add/2
  AeroDyn 3/1(Tau_r3) -> Add/3
  Beta_1/1 -> AeroDyn 1/3(Beta_1)
  Add/1 -> Tau_r/1
  Beta_2/1 -> AeroDyn 2/3(Beta_2)
  Beta_3/1 -> AeroDyn 3/3(Beta_3)
  v_w/1 -> Demux/1
  Demux/3 -> AeroDyn 3/1(v_w)
  Demux/2 -> AeroDyn 2/1(v_w)
  Demux/1 -> AeroDyn 1/1(v_w)

== system FDIBenchMark_BLW_test_b_1025/Controller/Subsystem ==
  Omega_g : Inport  OutDataType=sfix(16)  OutScaling=2^0
  Constant : Constant  Value=0  OutDataType=sfix(16)  OutScaling=2^0
  Gain : Gain  Gain=K_opt  ParameterDataType=sfix(16)  ParameterScaling=2^0  OutDataType=sfix(16)  OutScaling=2^0
  Product : Product  OutDataType=sfix(16)  OutScaling=2^0  RndMeth=Zero
  Beta_r : Outport  OutDataType=sfix(16)  OutScaling=2^0
  T_g,r : Outport  Port=2  OutDataType=sfix(16)  OutScaling=2^0
  wires:
  Constant/1 -> Beta_r/1
  Omega_g/1 -> Product/2, Product/1
  Gain/1 -> T_g,r/1
  Product/1 -> Gain/1

== system FDIBenchMark_BLW_test_b_1025/Controller/Subsystem1 ==
  P_r : Inport  OutDataType=sfix(16)  OutScaling=2^0
  Omega_g : Inport  Port=2  OutDataType=sfix(16)  OutScaling=2^0
  Add : Sum  OutDataType=sfix(16)  OutScaling=2^-10
  Bias : Bias  Bias=-Omega_nom
  Discrete-Time Integrator : DiscreteIntegrator  SampleTime=Ts  OutDataType=sfix(16)  OutScaling=2^0  LimitOutput=on  UpperSaturationLimit=90  LowerSaturationLimit=-2  ICPrevOutput=DiscIntNeverNeededParam  ICPrevScaledInput=DiscIntNeverNeededParam
  Divide : Product  Inputs=/*  OutDataType=sfix(16)  OutScaling=2^-10
  Gain : Gain  Gain=K_p  ParameterDataType=sfix(16)  ParameterScaling=2^0  OutDataType=sfix(16)  OutScaling=2^0
  Gain1 : Gain  Gain=K_i  ParameterDataType=sfix(16)  ParameterScaling=2^0  OutDataType=sfix(16)  OutScaling=2^0
  Gain2 : Gain  Gain=1/eta_gc  ParameterDataType=sfix(16)  ParameterScaling=2^0  OutDataType=sfix(16)  OutScaling=2^0
  Saturation : Saturate  UpperLimit=90  LowerLimit=-2  OutDataType=sfix(16)  OutScaling=2^0
  Beta_r : Outport  OutDataType=sfix(16)  OutScaling=2^0
  Tau_g,r : Outport  Port=2  OutDataType=sfix(16)  OutScaling=2^0
  wires:
  Divide/1 -> Gain2/1
  P_r/1 -> Divide/2
  Omega_g/1 -> Divide/1, Bias/1
  Bias/1 -> Discrete-Time Integrator/1, Gain/1
  Discrete-Time Integrator/1 -> Gain1/1
  Gain1/1 -> Add/2
  Gain/1 -> Add/1
  Add/1 -> Saturation/1
  Saturation/1 -> Beta_r/1
  Gain2/1 -> Tau_g,r/1

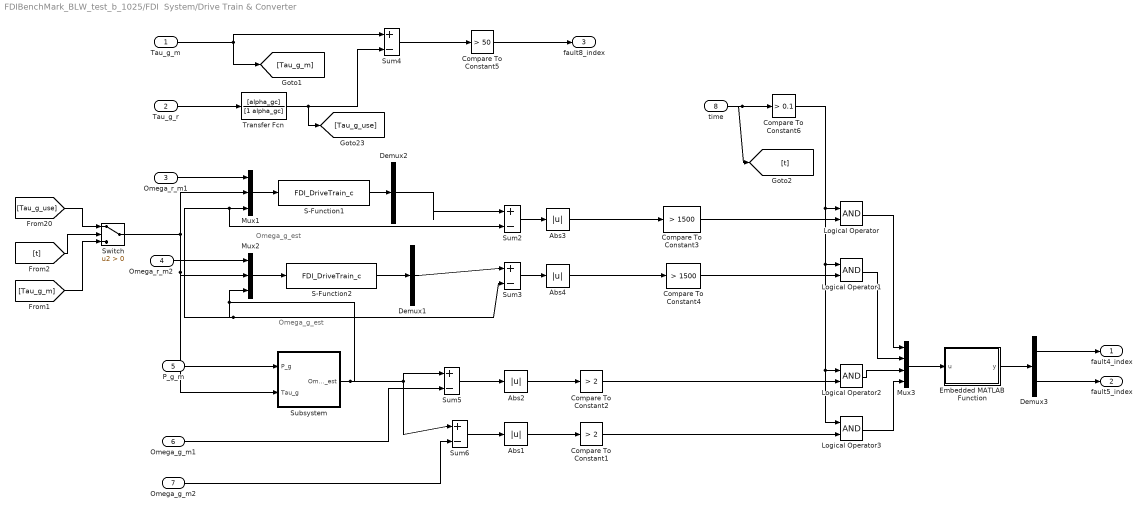
== system FDIBenchMark_BLW_test_b_1025/FDI  System/Drive Train & Converter ==
  note: Omega_g_est
  note: Omega_g_est
  Tau_g_m : Inport  OutDataType=fixdt(1, 16)  OutScaling=2^0
  Tau_g_r : Inport  Port=2  OutDataType=fixdt(1, 16)  OutScaling=2^0
  Omega_r_m1 : Inport  Port=3  OutDataType=fixdt(1, 16)  OutScaling=2^0
  Omega_r_m2 : Inport  Port=4  OutDataType=fixdt(1, 16)  OutScaling=2^0
  P_g_m : Inport  Port=5  OutDataType=fixdt(1, 16)  OutScaling=2^0
  Omega_g_m1 : Inport  Port=6  OutDataType=fixdt(1, 16)  OutScaling=2^0
  Omega_g_m2 : Inport  Port=7  OutDataType=fixdt(1, 16)  OutScaling=2^0
  time : Inport  Port=8  OutDataType=fixdt(1, 16)  OutScaling=2^0
  Abs{1..4} (4 alike) : Abs  ZeroCross=off  OutDataType=fixdt(1, 16)  OutScaling=2^0
  Compare To Constant1 : simulink/Logic and Bit Operations/Compare To Constant  SystemSampleTime=-1  relop=>  const=2  LogicOutDataTypeMode=uint8  ZeroCross=off
  Compare To Constant2 : simulink/Logic and Bit Operations/Compare To Constant  SystemSampleTime=-1  relop=>  const=2  LogicOutDataTypeMode=uint8  ZeroCross=off
  Compare To Constant3 : simulink/Logic and Bit Operations/Compare To Constant  SystemSampleTime=-1  relop=>  const=1500  LogicOutDataTypeMode=uint8  ZeroCross=off
  Compare To Constant4 : simulink/Logic and Bit Operations/Compare To Constant  SystemSampleTime=-1  relop=>  const=1500  LogicOutDataTypeMode=uint8  ZeroCross=off
  Compare To Constant5 : simulink/Logic and Bit Operations/Compare To Constant  SystemSampleTime=-1  relop=>  const=50  LogicOutDataTypeMode=uint8  ZeroCross=off
  Compare To Constant6 : simulink/Logic and Bit Operations/Compare To Constant  SystemSampleTime=-1  relop=>  const=0.1  LogicOutDataTypeMode=uint8  ZeroCross=off
  Demux1 : Demux  Outputs="[1  ]"
  Demux2 : Demux  Outputs="[1  ]"
  Demux3 : Demux  Outputs="[1  1]"
  Embedded MATLAB Function : Stateflow chart
  Logical Operator{,1..3} (4 alike) : Logic  AllPortsSameDT=off  OutDataTypeMode=boolean  LogicDataType=fixdt(0, 8)  OutDataTypeStr=boolean
  Mux1 : Mux  Inputs=3
  Mux2 : Mux  Inputs=3
  Mux3 : Mux
  S-Function1 : S-Function  FunctionName=FDI_DriveTrain_c  Parameters=A_DT, B_DT, C_DT, L_DT  EnableBusSupport=off
  S-Function2 : S-Function  FunctionName=FDI_DriveTrain_c  Parameters=A_DT, B_DT, C_DT, L_DT  EnableBusSupport=off
  Subsystem : Subsystem
  Sum{2..6} (5 alike) : Sum  Inputs=|+-  OutDataType=fixdt(1, 16)  OutScaling=2^0
  Switch : Switch  Criteria=u2 > Threshold  OutDataType=sfix(16)  OutScaling=2^0
  Transfer Fcn : TransferFcn  Numerator=[alpha_gc]  Denominator=[1 alpha_gc]
  fault4_index : Outport  OutDataType=fixdt(1, 16)  OutScaling=2^0
  fault5_index : Outport  Port=2  OutDataType=fixdt(1, 16)  OutScaling=2^0
  fault8_index : Outport  Port=3  OutDataType=fixdt(1, 16)  OutScaling=2^0
  wires:
  Mux1/1 -> S-Function1/1
  Demux2/1 -> Sum2/1
  S-Function1/1 -> Demux2/1
  Omega_r_m2/1 -> Mux2/1
  Mux2/1 -> S-Function2/1
  S-Function2/1 -> Demux1/1
  Tau_g_r/1 -> Transfer Fcn/1
  Transfer Fcn/1 -> Sum4/2, [Tau_g_use]
  Sum4/1 -> Compare To Constant5/1
  Tau_g_m/1 -> Sum4/1, [Tau_g_m]
  P_g_m/1 -> Subsystem/1(P_g)
  Omega_g_m1/1 -> Sum5/2
  Omega_g_m2/1 -> Sum6/2
  Demux1/1 -> Sum3/1
  Sum2/1 -> Abs3/1
  Sum3/1 -> Abs4/1
  Abs2/1 -> Compare To Constant2/1
  Sum5/1 -> Abs2/1
  Sum6/1 -> Abs1/1
  Abs1/1 -> Compare To Constant1/1
  Compare To Constant5/1 -> fault8_index/1
  Mux3/1 -> Embedded MATLAB Function/1(u)
  Demux3/1 -> fault4_index/1
  Demux3/2 -> fault5_index/1
  Embedded MATLAB Function/1(y) -> Demux3/1
  Abs4/1 -> Compare To Constant4/1
  Abs3/1 -> Compare To Constant3/1
  Omega_r_m1/1 -> Mux1/1
  Subsystem/1(Omega_g_est) -> Mux2/3, Sum3/2, Mux1/3, Sum2/2, Sum5/1, Sum6/1
  time/1 -> Compare To Constant6/1, [t]
  Compare To Constant6/1 -> Logical Operator/1, Logical Operator1/1, Logical Operator2/1, Logical Operator3/1
  Compare To Constant3/1 -> Logical Operator/2
  Logical Operator/1 -> Mux3/1
  Compare To Constant4/1 -> Logical Operator1/2
  Logical Operator1/1 -> Mux3/2
  Logical Operator2/1 -> Mux3/3
  Compare To Constant2/1 -> Logical Operator2/2
  Compare To Constant1/1 -> Logical Operator3/2
  Logical Operator3/1 -> Mux3/4
  [Tau_g_use] -> Switch/1
  [Tau_g_m] -> Switch/3
  [t] -> Switch/2
  Switch/1 -> Mux1/2, Mux2/2, Subsystem/2(Tau_g)

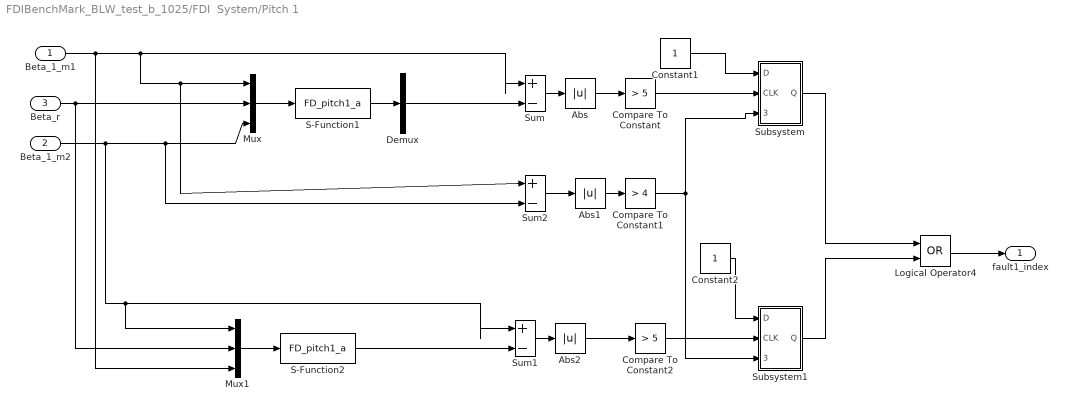
== system FDIBenchMark_BLW_test_b_1025/FDI  System/Pitch 1 ==
  Beta_1_m1 : Inport  OutDataType=fixdt(1, 16)  OutScaling=2^0
  Beta_1_m2 : Inport  Port=2  OutDataType=fixdt(1, 16)  OutScaling=2^0
  Beta_r : Inport  Port=3  OutDataType=fixdt(1, 16)  OutScaling=2^0
  Abs : Abs  ZeroCross=off  OutDataType=fixdt(1, 16)  OutScaling=2^0
  Abs1 : Abs  ZeroCross=off  OutDataType=fixdt(1, 16)  OutScaling=2^0
  Abs2 : Abs  ZeroCross=off  OutDataType=fixdt(1, 16)  OutScaling=2^0
  Compare To Constant : simulink/Logic and Bit Operations/Compare To Constant  SystemSampleTime=-1  relop=>  const=5  LogicOutDataTypeMode=uint8  ZeroCross=off
  Compare To Constant1 : simulink/Logic and Bit Operations/Compare To Constant  SystemSampleTime=-1  relop=>  const=4  LogicOutDataTypeMode=uint8  ZeroCross=off
  Compare To Constant2 : simulink/Logic and Bit Operations/Compare To Constant  SystemSampleTime=-1  relop=>  const=5  LogicOutDataTypeMode=uint8  ZeroCross=off
  Constant1 : Constant  OutDataType=fixdt(1, 16)  OutScaling=2^0
  Constant2 : Constant  OutDataType=fixdt(1, 16)  OutScaling=2^0
  Demux : Demux  Outputs="[1  ]"
  Logical Operator4 : Logic  Operator=OR  AllPortsSameDT=off  OutDataTypeMode=boolean  LogicDataType=fixdt(0, 8)  OutDataTypeStr=boolean
  Mux : Mux  Inputs=3
  Mux1 : Mux  Inputs=3
  S-Function1 : S-Function  FunctionName=FD_pitch1_a  Parameters=Apb_E,Bpb,Cpb,Lpb  EnableBusSupport=off
  S-Function2 : S-Function  FunctionName=FD_pitch1_a  Parameters=Apb_E,Bpb,Cpb,Lpb  EnableBusSupport=off
  Subsystem : Subsystem
  Subsystem1 : Subsystem
  Sum : Sum  Inputs=|+-  OutDataType=fixdt(1, 16)  OutScaling=2^0
  Sum1 : Sum  Inputs=|+-  OutDataType=fixdt(1, 16)  OutScaling=2^0
  Sum2 : Sum  Inputs=|+-  OutDataType=fixdt(1, 16)  OutScaling=2^0
  fault1_index : Outport  OutDataType=fixdt(1, 16)  OutScaling=2^0
  wires:
  Beta_1_m1/1 -> Mux/1, Sum2/1, Sum/1, Mux1/3
  Mux/1 -> S-Function1/1
  S-Function1/1 -> Demux/1
  Demux/1 -> Sum/2
  Beta_1_m2/1 -> Mux/3, Sum2/2, Mux1/1, Sum1/1
  Beta_r/1 -> Mux/2, Mux1/2
  Mux1/1 -> S-Function2/1
  S-Function2/1 -> Sum1/2
  Sum/1 -> Abs/1
  Abs/1 -> Compare To Constant/1
  Compare To Constant/1 -> Subsystem/2(CLK)
  Sum2/1 -> Abs1/1
  Abs1/1 -> Compare To Constant1/1
  Abs2/1 -> Compare To Constant2/1
  Compare To Constant2/1 -> Subsystem1/2(CLK)
  Sum1/1 -> Abs2/1
  Constant1/1 -> Subsystem/1(D)
  Constant2/1 -> Subsystem1/1(D)
  Subsystem/1(Q) -> Logical Operator4/1
  Subsystem1/1(Q) -> Logical Operator4/2
  Compare To Constant1/1 -> Subsystem/3(!CLR), Subsystem1/3(!CLR)
  Logical Operator4/1 -> fault1_index/1

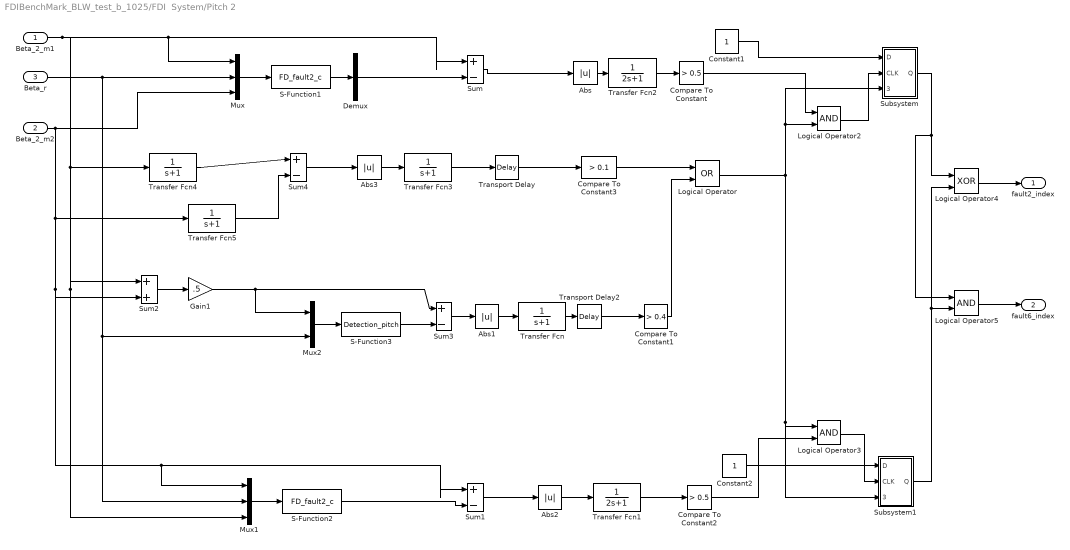
== system FDIBenchMark_BLW_test_b_1025/FDI  System/Pitch 2 ==
  Beta_2_m1 : Inport  OutDataType=fixdt(1, 16)  OutScaling=2^0
  Beta_2_m2 : Inport  Port=2  OutDataType=fixdt(1, 16)  OutScaling=2^0
  Beta_r : Inport  Port=3  OutDataType=fixdt(1, 16)  OutScaling=2^0
  Abs{,1..3} (4 alike) : Abs  ZeroCross=off  OutDataType=fixdt(1, 16)  OutScaling=2^0
  Compare To Constant : simulink/Logic and Bit Operations/Compare To Constant  SystemSampleTime=-1  relop=>  const=0.5  LogicOutDataTypeMode=uint8  ZeroCross=off
  Compare To Constant1 : simulink/Logic and Bit Operations/Compare To Constant  SystemSampleTime=-1  relop=>  const=0.4  LogicOutDataTypeMode=uint8  ZeroCross=off
  Compare To Constant2 : simulink/Logic and Bit Operations/Compare To Constant  SystemSampleTime=-1  relop=>  const=0.5  LogicOutDataTypeMode=uint8  ZeroCross=off
  Compare To Constant3 : simulink/Logic and Bit Operations/Compare To Constant  SystemSampleTime=-1  relop=>  const=0.1  LogicOutDataTypeMode=uint8  ZeroCross=off
  Constant1 : Constant  OutDataType=fixdt(1, 16)  OutScaling=2^0
  Constant2 : Constant  OutDataType=fixdt(1, 16)  OutScaling=2^0
  Demux : Demux  Outputs="[1  ]"
  Gain1 : Gain  Gain=.5  ParameterDataType=fixdt(1, 16)  ParameterScaling=2^0  OutDataType=fixdt(1, 16)  OutScaling=2^0
  Logical Operator : Logic  Operator=OR  AllPortsSameDT=off  OutDataTypeMode=boolean  LogicDataType=fixdt(0, 8)  OutDataTypeStr=boolean
  Logical Operator2 : Logic  AllPortsSameDT=off  OutDataTypeMode=boolean  LogicDataType=fixdt(0, 8)  OutDataTypeStr=boolean
  Logical Operator3 : Logic  AllPortsSameDT=off  OutDataTypeMode=boolean  LogicDataType=fixdt(0, 8)  OutDataTypeStr=boolean
  Logical Operator4 : Logic  Operator=XOR  AllPortsSameDT=off  OutDataTypeMode=boolean  LogicDataType=fixdt(0, 8)  OutDataTypeStr=boolean
  Logical Operator5 : Logic  AllPortsSameDT=off  OutDataTypeMode=boolean  LogicDataType=fixdt(0, 8)  OutDataTypeStr=boolean
  Mux : Mux  Inputs=3
  Mux1 : Mux  Inputs=3
  Mux2 : Mux  Inputs=2
  S-Function1 : S-Function  FunctionName=FD_fault2_c  Parameters=Apb_E,Bpb,Cpb,Lpb  EnableBusSupport=off
  S-Function2 : S-Function  FunctionName=FD_fault2_c  Parameters=Apb_E,Bpb,Cpb,Lpb  EnableBusSupport=off
  S-Function3 : S-Function  FunctionName=Detection_pitch  Parameters=Apb,Bpb,Cpb,Lpb_FD  EnableBusSupport=off
  Subsystem : Subsystem
  Subsystem1 : Subsystem
  Sum{,1,3..4} (4 alike) : Sum  Inputs=|+-  OutDataType=fixdt(1, 16)  OutScaling=2^0
  Sum2 : Sum  Inputs=|++  OutDataType=fixdt(1, 16)  OutScaling=2^0
  Transfer Fcn : TransferFcn  Denominator=[1 1]
  Transfer Fcn1 : TransferFcn  Denominator="[2  1]"
  Transfer Fcn2 : TransferFcn  Denominator="[2  1]"
  Transfer Fcn3 : TransferFcn  Denominator=[1 1]
  Transfer Fcn4 : TransferFcn  Denominator="[1  1]"
  Transfer Fcn5 : TransferFcn  Denominator="[1  1]"
  Transport Delay : TransportDelay  DelayTime=0.5
  Transport Delay2 : TransportDelay  DelayTime=0.5
  fault2_index : Outport  OutDataType=fixdt(1, 16)  OutScaling=2^0
  fault6_index : Outport  Port=2  OutDataType=fixdt(1, 16)  OutScaling=2^0
  wires:
  Logical Operator5/1 -> fault6_index/1
  Logical Operator4/1 -> fault2_index/1
  Abs3/1 -> Transfer Fcn3/1
  Transfer Fcn3/1 -> Transport Delay/1
  Transfer Fcn5/1 -> Sum4/2
  Transfer Fcn4/1 -> Sum4/1
  Logical Operator3/1 -> Subsystem1/2(CLK)
  Gain1/1 -> Mux2/1, Sum3/1
  Sum2/1 -> Gain1/1
  Compare To Constant/1 -> Logical Operator2/1
  Logical Operator2/1 -> Subsystem/2(CLK)
  Transfer Fcn1/1 -> Compare To Constant2/1
  Abs2/1 -> Transfer Fcn1/1
  Sum1/1 -> Abs2/1
  Transfer Fcn2/1 -> Compare To Constant/1
  Abs/1 -> Transfer Fcn2/1
  Transfer Fcn/1 -> Transport Delay2/1
  Abs1/1 -> Transfer Fcn/1
  Subsystem1/1(Q) -> Logical Operator4/2, Logical Operator5/2
  Constant2/1 -> Subsystem1/1(D)
  Compare To Constant2/1 -> Logical Operator3/2
  Logical Operator/1 -> Subsystem/3(!CLR), Logical Operator2/2, Subsystem1/3(!CLR), Logical Operator3/1
  Subsystem/1(Q) -> Logical Operator4/1, Logical Operator5/1
  Constant1/1 -> Subsystem/1(D)
  Compare To Constant1/1 -> Logical Operator/2
  Compare To Constant3/1 -> Logical Operator/1
  Sum4/1 -> Abs3/1
  Sum3/1 -> Abs1/1
  S-Function3/1 -> Sum3/2
  Mux2/1 -> S-Function3/1
  Sum/1 -> Abs/1
  S-Function2/1 -> Sum1/2
  Mux1/1 -> S-Function2/1
  Demux/1 -> Sum/2
  S-Function1/1 -> Demux/1
  Mux/1 -> S-Function1/1
  Beta_2_m1/1 -> Mux/1, Sum/1, Transfer Fcn4/1, Sum2/1, Mux1/3
  Beta_2_m2/1 -> Mux/3, Transfer Fcn5/1, Sum2/2, Mux1/1, Sum1/1
  Beta_r/1 -> Mux/2, Mux2/2, Mux1/2
  Transport Delay/1 -> Compare To Constant3/1
  Transport Delay2/1 -> Compare To Constant1/1

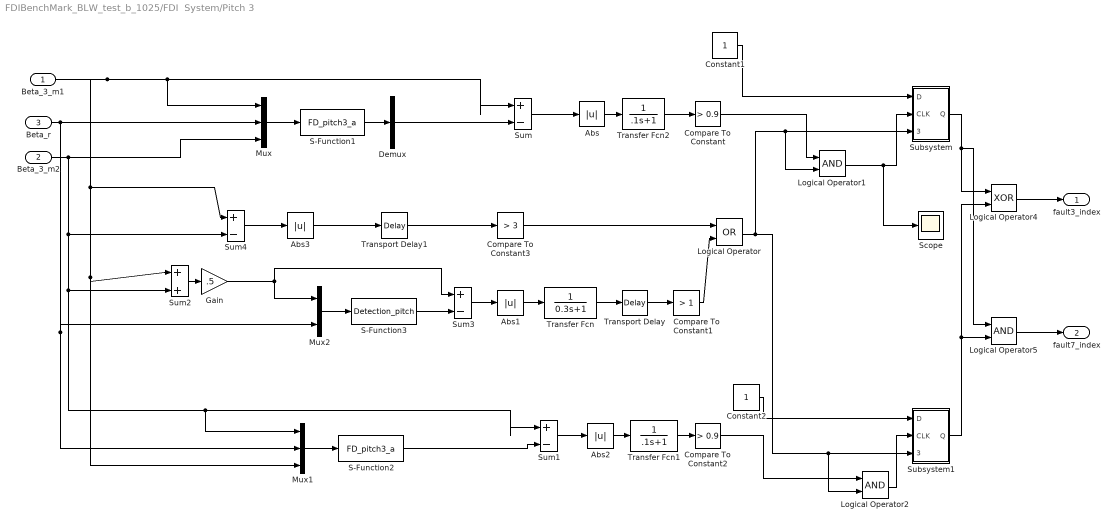
== system FDIBenchMark_BLW_test_b_1025/FDI  System/Pitch 3 ==
  Beta_3_m1 : Inport  OutDataType=fixdt(1, 16)  OutScaling=2^0
  Beta_3_m2 : Inport  Port=2  OutDataType=fixdt(1, 16)  OutScaling=2^0
  Beta_r : Inport  Port=3  OutDataType=fixdt(1, 16)  OutScaling=2^0
  Abs{,1..3} (4 alike) : Abs  ZeroCross=off  OutDataType=fixdt(1, 16)  OutScaling=2^0
  Compare To Constant : simulink/Logic and Bit Operations/Compare To Constant  SystemSampleTime=-1  relop=>  const=0.9  LogicOutDataTypeMode=uint8  ZeroCross=off
  Compare To Constant1 : simulink/Logic and Bit Operations/Compare To Constant  SystemSampleTime=-1  relop=>  const=1  LogicOutDataTypeMode=uint8  ZeroCross=off
  Compare To Constant2 : simulink/Logic and Bit Operations/Compare To Constant  SystemSampleTime=-1  relop=>  const=0.9  LogicOutDataTypeMode=uint8  ZeroCross=off
  Compare To Constant3 : simulink/Logic and Bit Operations/Compare To Constant  SystemSampleTime=-1  relop=>  const=3  LogicOutDataTypeMode=uint8  ZeroCross=off
  Constant1 : Constant  OutDataType=fixdt(1, 16)  OutScaling=2^0
  Constant2 : Constant  OutDataType=fixdt(1, 16)  OutScaling=2^0
  Demux : Demux  Outputs="[1  ]"
  Gain : Gain  Gain=.5  ParameterDataType=fixdt(1, 16)  ParameterScaling=2^0  OutDataType=fixdt(1, 16)  OutScaling=2^0
  Logical Operator : Logic  Operator=OR  AllPortsSameDT=off  OutDataTypeMode=boolean  LogicDataType=fixdt(0, 8)  OutDataTypeStr=boolean
  Logical Operator1 : Logic  AllPortsSameDT=off  OutDataTypeMode=boolean  LogicDataType=fixdt(0, 8)  OutDataTypeStr=boolean
  Logical Operator2 : Logic  AllPortsSameDT=off  OutDataTypeMode=boolean  LogicDataType=fixdt(0, 8)  OutDataTypeStr=boolean
  Logical Operator4 : Logic  Operator=XOR  AllPortsSameDT=off  OutDataTypeMode=boolean  LogicDataType=fixdt(0, 8)  OutDataTypeStr=boolean
  Logical Operator5 : Logic  AllPortsSameDT=off  OutDataTypeMode=boolean  LogicDataType=fixdt(0, 8)  OutDataTypeStr=boolean
  Mux : Mux  Inputs=3
  Mux1 : Mux  Inputs=3
  Mux2 : Mux  Inputs=2
  S-Function1 : S-Function  FunctionName=FD_pitch3_a  Parameters=Apb_E,Bpb,Cpb,Lpb  EnableBusSupport=off
  S-Function2 : S-Function  FunctionName=FD_pitch3_a  Parameters=Apb_E,Bpb,Cpb,Lpb  EnableBusSupport=off
  S-Function3 : S-Function  FunctionName=Detection_pitch  Parameters=Apb,Bpb,Cpb,Lpb_FD  EnableBusSupport=off
  Scope : Scope
      settings: SaveName=S
  Subsystem : Subsystem
  Subsystem1 : Subsystem
  Sum{,1,3..4} (4 alike) : Sum  Inputs=|+-  OutDataType=fixdt(1, 16)  OutScaling=2^0
  Sum2 : Sum  Inputs=|++  OutDataType=fixdt(1, 16)  OutScaling=2^0
  Transfer Fcn : TransferFcn  Denominator=[0.3 1]
  Transfer Fcn1 : TransferFcn  Denominator=[.1 1]
  Transfer Fcn2 : TransferFcn  Denominator=[.1 1]
  Transport Delay : TransportDelay  DelayTime=0.5
  Transport Delay1 : TransportDelay  DelayTime=0.5
  fault3_index : Outport  OutDataType=fixdt(1, 16)  OutScaling=2^0
  fault7_index : Outport  Port=2  OutDataType=fixdt(1, 16)  OutScaling=2^0
  wires:
  Logical Operator5/1 -> fault7_index/1
  Logical Operator4/1 -> fault3_index/1
  Abs3/1 -> Transport Delay1/1
  Logical Operator2/1 -> Subsystem1/2(CLK)
  Compare To Constant2/1 -> Logical Operator2/1
  Logical Operator1/1 -> Subsystem/2(CLK), Scope/1
  Compare To Constant/1 -> Logical Operator1/1
  Transfer Fcn2/1 -> Compare To Constant/1
  Transfer Fcn1/1 -> Compare To Constant2/1
  Compare To Constant3/1 -> Logical Operator/1
  Logical Operator/1 -> Subsystem/3(!CLR), Logical Operator1/2, Subsystem1/3(!CLR), Logical Operator2/2
  Abs1/1 -> Transfer Fcn/1
  Sum4/1 -> Abs3/1
  Sum/1 -> Abs/1
  Subsystem/1(Q) -> Logical Operator4/1, Logical Operator5/1
  Constant1/1 -> Subsystem/1(D)
  Abs/1 -> Transfer Fcn2/1
  Beta_r/1 -> Mux/2, Mux1/2, Mux2/2
  Beta_3_m2/1 -> Mux/3, Sum2/2, Mux1/1, Sum1/1, Sum4/2
  Demux/1 -> Sum/2
  S-Function1/1 -> Demux/1
  Mux/1 -> S-Function1/1
  Beta_3_m1/1 -> Mux/1, Sum/1, Sum2/1, Mux1/3, Sum4/1
  Subsystem1/1(Q) -> Logical Operator4/2, Logical Operator5/2
  Constant2/1 -> Subsystem1/1(D)
  Abs2/1 -> Transfer Fcn1/1
  Sum1/1 -> Abs2/1
  S-Function2/1 -> Sum1/2
  Mux1/1 -> S-Function2/1
  Sum2/1 -> Gain/1
  Gain/1 -> Mux2/1, Sum3/1
  Sum3/1 -> Abs1/1
  S-Function3/1 -> Sum3/2
  Mux2/1 -> S-Function3/1
  Compare To Constant1/1 -> Logical Operator/2
  Transfer Fcn/1 -> Transport Delay/1
  Transport Delay/1 -> Compare To Constant1/1
  Transport Delay1/1 -> Compare To Constant3/1

== system FDIBenchMark_BLW_test_b_1025/Sensors/Omega_g Sensor ==
  Omega_g : Inport
  Fault_5 : Inport  Port=2
  Add : Sum  OutDataType=sfix(16)  OutScaling=2^-10
  Add1 : Sum  OutDataType=sfix(16)  OutScaling=2^-10
  Band-Limited White Noise : simulink/Sources/Band-Limited White Noise  SystemSampleTime=-1  Cov=Np_omega_g  Ts=Ts  seed=seed(4)
  Band-Limited White Noise1 : simulink/Sources/Band-Limited White Noise  SystemSampleTime=-1  Cov=Np_omega_g  Ts=Ts  seed=seed(5)
  Gain : Gain  Gain=Gain_Omega_r_m2  ParameterDataType=sfix(16)  ParameterScaling=2^0  OutDataType=sfix(16)  OutScaling=2^0
  Switch1 : Switch  Threshold=0.5  OutDataType=sfix(16)  OutScaling=2^0
  Omega_g_m1 : Outport
  Omega_g_m2 : Outport  Port=2
  wires:
  Band-Limited White Noise1/1 -> Add1/2
  Band-Limited White Noise/1 -> Add/1
  Omega_g/1 -> Add1/1, Add/2
  Add/1 -> Omega_g_m1/1
  Add1/1 -> Switch1/1, Gain/1
  Switch1/1 -> Omega_g_m2/1
  Fault_5/1 -> Switch1/2
  Gain/1 -> Switch1/3

== system FDIBenchMark_BLW_test_b_1025/Sensors/Omega_r Sensor ==
  Omega_r : Inport
  Fault_4 : Inport  Port=2
  Fault_5 : Inport  Port=3
  Add : Sum  OutDataType=sfix(16)  OutScaling=2^-10
  Add1 : Sum  OutDataType=sfix(16)  OutScaling=2^-10
  Band-Limited White Noise : simulink/Sources/Band-Limited White Noise  SystemSampleTime=-1  Cov=Np_omega_r  Ts=Ts  seed=seed(2)
  Band-Limited White Noise1 : simulink/Sources/Band-Limited White Noise  SystemSampleTime=-1  Cov=Np_omega_r  Ts=Ts  seed=seed(3)
  Constant : Constant  Value=Constant_Omega_r_m1  OutDataType=sfix(16)  OutScaling=2^0
  Gain : Gain  Gain=Gain_Omega_r_m2  ParameterDataType=sfix(16)  ParameterScaling=2^0  OutDataType=sfix(16)  OutScaling=2^0
  Switch : Switch  Threshold=0.5  OutDataType=sfix(16)  OutScaling=2^0
  Switch1 : Switch  Threshold=0.5  OutDataType=sfix(16)  OutScaling=2^0
  Omega_r_m1 : Outport
  Omega_r_m2 : Outport  Port=2
  wires:
  Omega_r/1 -> Add/2, Add1/1
  Band-Limited White Noise/1 -> Add/1
  Band-Limited White Noise1/1 -> Add1/2
  Fault_4/1 -> Switch/2
  Constant/1 -> Switch/3
  Add/1 -> Switch/1
  Switch/1 -> Omega_r_m1/1
  Add1/1 -> Switch1/1, Gain/1
  Switch1/1 -> Omega_r_m2/1
  Fault_5/1 -> Switch1/2
  Gain/1 -> Switch1/3

== system FDIBenchMark_BLW_test_b_1025/Sensors/P_g Sensor ==
  P_g : Inport
  Add : Sum  OutDataType=sfix(16)  OutScaling=2^-10
  Band-Limited White Noise : simulink/Sources/Band-Limited White Noise  SystemSampleTime=-1  Cov=Np_P_g  Ts=Ts  seed=seed(7)
  P_g_m : Outport
  wires:
  Band-Limited White Noise/1 -> Add/2
  P_g/1 -> Add/1
  Add/1 -> P_g_m/1

== system FDIBenchMark_BLW_test_b_1025/Sensors/Pitch1 Sensor ==
  Beta_1 : Inport
  Fault_1 : Inport  Port=2
  Add : Sum  OutDataType=sfix(16)  OutScaling=2^-10
  Add1 : Sum  OutDataType=sfix(16)  OutScaling=2^-10
  Band-Limited White Noise : simulink/Sources/Band-Limited White Noise  SystemSampleTime=-1  Cov=Np_beta  Ts=Ts  seed=seed(8)
  Band-Limited White Noise1 : simulink/Sources/Band-Limited White Noise  SystemSampleTime=-1  Cov=Np_beta  Ts=Ts  seed=seed(9)
  Constant : Constant  Value=Constant_Beta_1_m1  OutDataType=sfix(16)  OutScaling=2^0
  Switch : Switch  Threshold=0.5  OutDataType=sfix(16)  OutScaling=2^0
  Beta_1_m1 : Outport
  Beta_1_m2 : Outport  Port=2
  wires:
  Band-Limited White Noise1/1 -> Add1/2
  Add1/1 -> Beta_1_m2/1
  Band-Limited White Noise/1 -> Add/1
  Beta_1/1 -> Add1/1, Add/2
  Fault_1/1 -> Switch/2
  Constant/1 -> Switch/3
  Add/1 -> Switch/1
  Switch/1 -> Beta_1_m1/1

== system FDIBenchMark_BLW_test_b_1025/Sensors/Pitch2 Sensor ==
  Beta_2 : Inport
  Fault_2 : Inport  Port=2
  Add : Sum  OutDataType=sfix(16)  OutScaling=2^-10
  Add1 : Sum  OutDataType=sfix(16)  OutScaling=2^-10
  Band-Limited White Noise : simulink/Sources/Band-Limited White Noise  SystemSampleTime=-1  Cov=Np_beta  Ts=Ts  seed=seed(10)
  Band-Limited White Noise1 : simulink/Sources/Band-Limited White Noise  SystemSampleTime=-1  Cov=Np_beta  Ts=Ts  seed=seed(11)
  Gain : Gain  Gain=Gain_Beta_2_m2  ParameterDataType=sfix(16)  ParameterScaling=2^0  OutDataType=sfix(16)  OutScaling=2^0
  Switch : Switch  Threshold=.5  OutDataType=sfix(16)  OutScaling=2^0
  Beta_2_m1 : Outport
  Beta_2_m2 : Outport  Port=2
  wires:
  Band-Limited White Noise1/1 -> Add1/2
  Band-Limited White Noise/1 -> Add/1
  Beta_2/1 -> Add1/1, Add/2
  Add/1 -> Beta_2_m1/1
  Add1/1 -> Switch/1, Gain/1
  Gain/1 -> Switch/3
  Switch/1 -> Beta_2_m2/1
  Fault_2/1 -> Switch/2

== system FDIBenchMark_BLW_test_b_1025/Sensors/Pitch3 Sensor ==
  Beta_3 : Inport
  Fault_3 : Inport  Port=2
  Add : Sum  OutDataType=sfix(16)  OutScaling=2^-10
  Add1 : Sum  OutDataType=sfix(16)  OutScaling=2^-10
  Band-Limited White Noise1 : simulink/Sources/Band-Limited White Noise  SystemSampleTime=-1  Cov=Np_beta  Ts=Ts  seed=seed(13)
  Band-Limited White Noise2 : simulink/Sources/Band-Limited White Noise  SystemSampleTime=-1  Cov=Np_beta  Ts=Ts  seed=seed(12)
  Constant : Constant  Value=Constant_Beta_3_m1  OutDataType=sfix(16)  OutScaling=2^0
  Switch : Switch  Threshold=0.5  OutDataType=sfix(16)  OutScaling=2^0
  Beta_3_m1 : Outport
  Beta_3_m2 : Outport  Port=2
  wires:
  Band-Limited White Noise1/1 -> Add1/2
  Add1/1 -> Beta_3_m2/1
  Band-Limited White Noise2/1 -> Add/1
  Beta_3/1 -> Add1/1, Add/2
  Fault_3/1 -> Switch/2
  Constant/1 -> Switch/3
  Add/1 -> Switch/1
  Switch/1 -> Beta_3_m1/1

== system FDIBenchMark_BLW_test_b_1025/Sensors/Tau_g Sensor ==
  Tau_g : Inport
  Add : Sum  OutDataType=sfix(16)  OutScaling=2^-10
  Band-Limited White Noise : simulink/Sources/Band-Limited White Noise  SystemSampleTime=-1  Cov=Np_tau_g  Ts=Ts  seed=seed(6)
  Tau_g_m : Outport
  wires:
  Add/1 -> Tau_g_m/1
  Tau_g/1 -> Add/1
  Band-Limited White Noise/1 -> Add/2
